simulink model "Simulink_Model"  (R2021a)
settings: Solver=VariableStepAuto  StartTime=0.0  StopTime=10.0  RelTol=1e-3
libraries: cstblocks x2
settings Model: Creator=Euge Etcheverry  LastModifiedBy=Euge Etcheverry

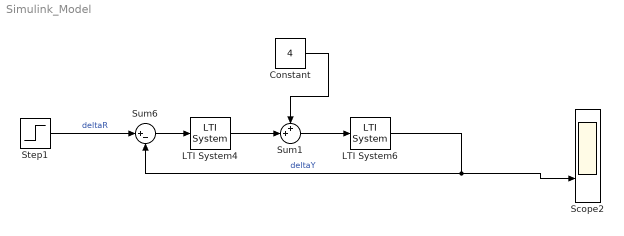
== system Simulink_Model ==
  Constant : Constant  Value=4
  LTI System4 : cstblocks/LTI System  sys=Cd  IC=[]
  LTI System6 : cstblocks/LTI System  sys=P  IC=[]
  Scope2 : Scope  NumInputPorts=2
  Step1 : Step  After=1.5  SampleTime=0
  Sum1 : Sum  Inputs=++|
  Sum6 : Sum  Inputs=|+-
  wires:
  Step1/1 -> Sum6/1  "deltaR"
  Constant/1 -> Sum1/1
  Sum6/1 -> LTI System4/1
  LTI System4/1 -> Sum1/2
  Sum1/1 -> LTI System6/1
  LTI System6/1 -> Sum6/2, Scope2/2  "deltaY"
